simulink model "main_simulation_without_Fw"  (R2015a)
settings: Solver=ode5  StartTime=0.0  StopTime=10  FixedStep=5e-4  RelTol=1e-3
values from neighbouring files (symbols this model uses):
  A = [125.649383136 -1075.44985766 0 0 236.024000906 -128.804687365 0 0 0 0 92.6500650057 -307.515794138 ... (16 elements, 4x4)]    [A.mat]
  B = [-913.807005742  410.133075183; -1063.47882704  330.077603124; 226.197070552  159.639712061; -293.138793165  -247.710273712]    [B.mat]
  C = [-0.0510975239854  0.0401880943917  -0.0900037144493  -0.119486841348; 0.0203356964471  -0.016074315274  -0.0637171533365  -0.0826343516286]    [C.mat]
  H = [329.317967573 -1053.24967937 -858.225293938 -252.074170822]    [H.mat]
  K = [0  0  0  0; 0  0  0  0]    [K.mat]
  Kw = [0 0]    [Kw.mat]
  L = [0 0 0]    [L.mat]
undefined symbols (not defined in the file or in its folder): At2, Bt2, Ct, Gt2, Ht, Q1, Qbx, Qby, R, Sai1, Sai2, Sai3, Sai4, Sigma1
libraries: simulink x3
settings Model: Creator=p4wp4w  LastModifiedBy=p4wp4w

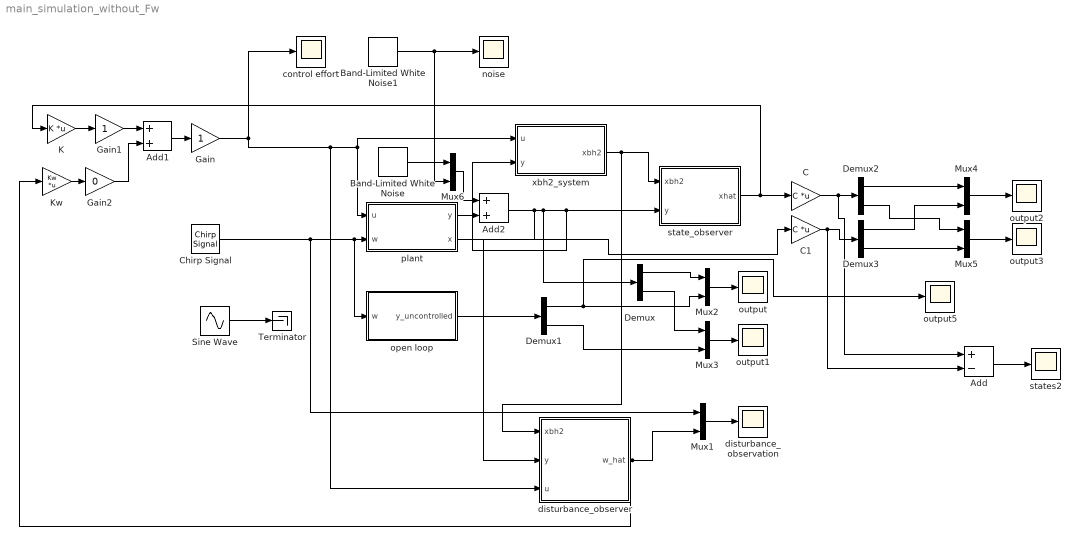
== system main_simulation_without_Fw ==
  Add : Sum  Inputs=+-
  Add1 : Sum
  Add2 : Sum
  Band-Limited White Noise : simulink/Sources/Band-Limited White Noise  Cov=[0.000001]  Ts=5e-4  seed=[23341]
  Band-Limited White Noise1 : simulink/Sources/Band-Limited White Noise  Cov=[0.000001]  Ts=5e-4  seed=[23341]
  C : Gain  Gain=C  Multiplication=Matrix(K*u)
  C1 : Gain  Gain=C  Multiplication=Matrix(K*u)
  Chirp Signal : simulink/Sources/Chirp Signal  f1=0.1  T=10  f2=85
  Demux{,1..3} (4 alike) : Demux  Outputs=2
  Gain : Gain
  Gain1 : Gain
  Gain2 : Gain  Gain=0
  K : Gain  Gain=K  Multiplication=Matrix(K*u)
  Kw : Gain  Gain=Kw  Multiplication=Matrix(K*u)
  Mux{1..6} (6 alike) : Mux  Inputs=2
  Sine Wave : Sin  Frequency=14*2*pi  SampleTime=0
  Terminator : Terminator
  "control effort " : Scope
      settings: SaveName=ScopeData5
  disturbance_observation : Scope
      settings: SaveName=ScopeData4
  disturbance_observer : Subsystem
  noise : Scope
      settings: YMin=-0.55  YMax=0.5  SaveName=ScopeData8
  open loop : Subsystem
  output{,1..3,5} (5 alike) : Scope
      output settings: YMin=-30  YMax=30
      output2 settings: YMin=-1.75  YMax=1.5  SaveName=ScopeData2
      output3 settings: SaveName=ScopeData3
      output5 settings: SaveName=ScopeData6
  plant : Subsystem
  state_observer : Subsystem
  states2 : Scope
      settings: SaveName=ScopeData7
  xbh2_system : Subsystem
  wires:
  Chirp Signal/1 -> Mux1/1, open loop/1(w), plant/2(w)
  state_observer/1(xhat) -> K/1, C/1
  plant/2(x) -> C1/1
  xbh2_system/1(xbh2) -> disturbance_observer/1(xbh2), state_observer/1(xbh2)
  Mux1/1 -> disturbance_observation/1
  disturbance_observer/1(w_hat) -> Kw/1, Mux1/2
  Mux2/1 -> output/1
  Mux3/1 -> output1/1
  Demux/1 -> Mux2/1
  Demux/2 -> Mux3/1
  open loop/1(y_uncontrolled) -> Demux1/1
  Demux1/1 -> output5/1, Mux2/2
  Demux1/2 -> Mux3/2
  Gain/1 -> disturbance_observer/3(u), plant/1(u), xbh2_system/1(u), "control effort "/1
  C/1 -> Add/1, Demux2/1
  C1/1 -> Add/2, Demux3/1
  Demux2/1 -> Mux4/1
  Demux3/1 -> Mux4/2
  Demux2/2 -> Mux5/1
  Demux3/2 -> Mux5/2
  Mux4/1 -> output2/1
  Mux5/1 -> output3/1
  Add/1 -> states2/1
  Sine Wave/1 -> Terminator/1
  Add1/1 -> Gain/1
  K/1 -> Gain1/1
  Gain1/1 -> Add1/1
  Gain2/1 -> Add1/2
  Kw/1 -> Gain2/1
  plant/1(y) -> Add2/2
  Band-Limited White Noise/1 -> Mux6/1
  Mux6/1 -> Add2/1
  Band-Limited White Noise1/1 -> noise/1, Mux6/2
  Add2/1 -> disturbance_observer/2(y), Demux/1, xbh2_system/2(y), state_observer/2(y)

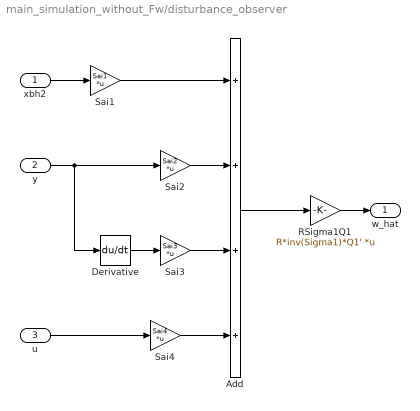
== system main_simulation_without_Fw/disturbance_observer ==
  xbh2 : Inport
  y : Inport  Port=2
  u : Inport  Port=3
  Add : Sum  Inputs=++++
  Derivative : Derivative
  RSigma1Q1 : Gain  Gain=R*inv(Sigma1)*Q1'  Multiplication=Matrix(K*u)
  Sai1 : Gain  Gain=Sai1  Multiplication=Matrix(K*u)
  Sai2 : Gain  Gain=Sai2  Multiplication=Matrix(K*u)
  Sai3 : Gain  Gain=Sai3  Multiplication=Matrix(K*u)
  Sai4 : Gain  Gain=Sai4  Multiplication=Matrix(K*u)
  w_hat : Outport
  wires:
  RSigma1Q1/1 -> w_hat/1
  Add/1 -> RSigma1Q1/1
  Sai1/1 -> Add/1
  Sai2/1 -> Add/2
  Sai3/1 -> Add/3
  Sai4/1 -> Add/4
  xbh2/1 -> Sai1/1
  y/1 -> Derivative/1, Sai2/1
  Derivative/1 -> Sai3/1
  u/1 -> Sai4/1

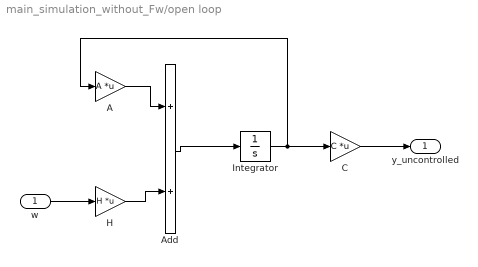
== system main_simulation_without_Fw/open loop ==
  w : Inport
  A : Gain  Gain=A  Multiplication=Matrix(K*u)
  Add : Sum
  C : Gain  Gain=C  Multiplication=Matrix(K*u)
  H : Gain  Gain=H  Multiplication=Matrix(K*u)
  Integrator : Integrator
  y_uncontrolled : Outport
  wires:
  C/1 -> y_uncontrolled/1
  H/1 -> Add/2
  A/1 -> Add/1
  Integrator/1 -> A/1, C/1
  Add/1 -> Integrator/1
  w/1 -> H/1

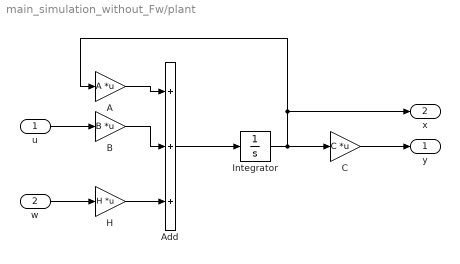
== system main_simulation_without_Fw/plant ==
  u : Inport
  w : Inport  Port=2
  A : Gain  Gain=A  Multiplication=Matrix(K*u)
  Add : Sum  Inputs=+++
  B : Gain  Gain=B  Multiplication=Matrix(K*u)
  C : Gain  Gain=C  Multiplication=Matrix(K*u)
  H : Gain  Gain=H  Multiplication=Matrix(K*u)
  Integrator : Integrator
  y : Outport
  x : Outport  Port=2
  wires:
  w/1 -> H/1
  u/1 -> B/1
  Add/1 -> Integrator/1
  B/1 -> Add/2
  Integrator/1 -> C/1, x/1, A/1
  A/1 -> Add/1
  H/1 -> Add/3
  C/1 -> y/1

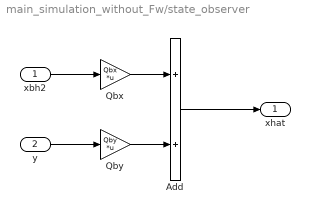
== system main_simulation_without_Fw/state_observer ==
  xbh2 : Inport
  y : Inport  Port=2
  Add : Sum
  Qbx : Gain  Gain=Qbx  Multiplication=Matrix(K*u)
  Qby : Gain  Gain=Qby  Multiplication=Matrix(K*u)
  xhat : Outport
  wires:
  Add/1 -> xhat/1
  y/1 -> Qby/1
  xbh2/1 -> Qbx/1
  Qby/1 -> Add/2
  Qbx/1 -> Add/1

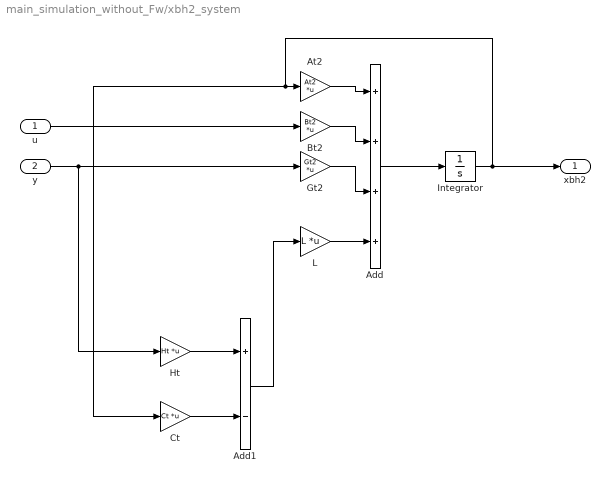
== system main_simulation_without_Fw/xbh2_system ==
  u : Inport
  y : Inport  Port=2
  Add : Sum  Inputs=++++
  Add1 : Sum  Inputs=+-
  At2 : Gain  Gain=At2  Multiplication=Matrix(K*u)
  Bt2 : Gain  Gain=Bt2  Multiplication=Matrix(K*u)
  Ct : Gain  Gain=Ct  Multiplication=Matrix(K*u)
  Gt2 : Gain  Gain=Gt2  Multiplication=Matrix(K*u)
  Ht : Gain  Gain=Ht  Multiplication=Matrix(K*u)
  Integrator : Integrator
  L : Gain  Gain=L  Multiplication=Matrix(K*u)
  xbh2 : Outport
  wires:
  Gt2/1 -> Add/3
  At2/1 -> Add/1
  Integrator/1 -> xbh2/1, At2/1, Ct/1
  Bt2/1 -> Add/2
  Add/1 -> Integrator/1
  u/1 -> Bt2/1
  y/1 -> Ht/1, Gt2/1
  L/1 -> Add/4
  Ct/1 -> Add1/2
  Add1/1 -> L/1
  Ht/1 -> Add1/1
